simulink model "pendulum_2"  (R2013b)
settings: Solver=ode45  StartTime=0.0  StopTime=10.0  RelTol=1e-3
undefined symbols (not defined in the file or in its folder): g, l_p, l_w, m_car, v_R
settings Model: Creator=daniel  LastModifiedBy=daniel

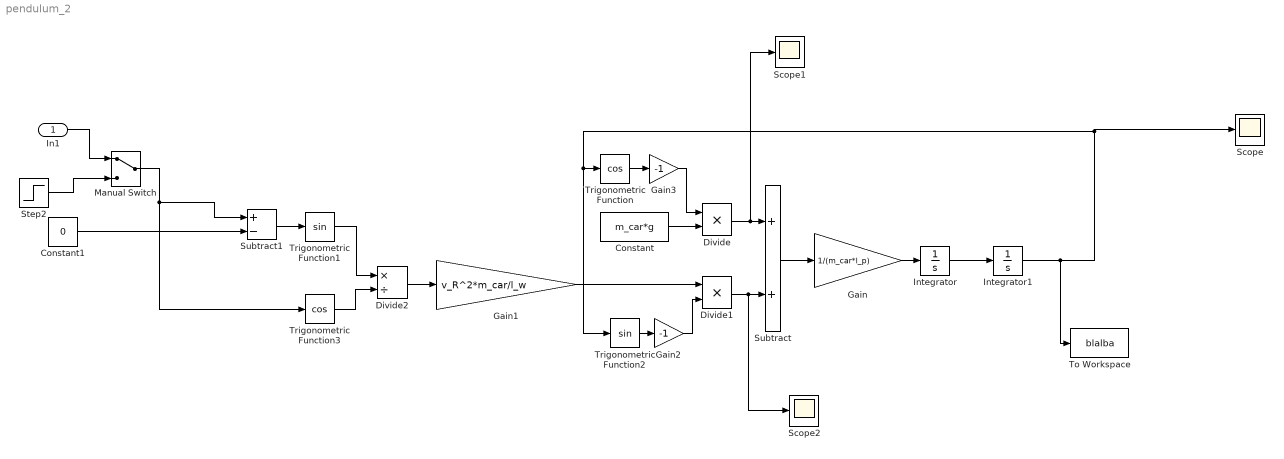
== system pendulum_2 ==
  In1 : Inport
  Constant : Constant  Value=m_car*g
  Constant1 : Constant  Value=0
  Divide : Product  Inputs=**
  Divide1 : Product  Inputs=**
  Divide2 : Product  Inputs=*/
  Gain : Gain  Gain=1/(m_car*l_p)
  Gain1 : Gain  Gain=v_R^2*m_car/l_w
  Gain2 : Gain  Gain=-1
  Gain3 : Gain  Gain=-1
  Integrator : Integrator  ContinuousStateAttributes='rho_dot'
  Integrator1 : Integrator  InitialCondition=pi/2+0.01  ContinuousStateAttributes='rho'
  Manual Switch : ManualSwitch
  Scope : Scope
  Scope1 : Scope
  Scope2 : Scope
      settings: SaveName=ScopeData2
  Step2 : Step  Time=7  After=0.8  SampleTime=0.01
  Subtract : Sum
  Subtract1 : Sum  Inputs=+-
  To Workspace : ToWorkspace  VariableName=blalba  SampleTime=-1  SaveFormat=Timeseries
  Trigonometric Function : Trigonometry  Operator=cos
  Trigonometric Function1 : Trigonometry
  Trigonometric Function2 : Trigonometry
  Trigonometric Function3 : Trigonometry  Operator=cos
  wires:
  Integrator/1 -> Integrator1/1
  Divide1/1 -> Scope2/1, Subtract/2
  Divide/1 -> Scope1/1, Subtract/1
  Manual Switch/1 -> Trigonometric Function3/1, Subtract1/1
  Constant1/1 -> Subtract1/2
  Trigonometric Function1/1 -> Divide2/1
  Trigonometric Function/1 -> Gain3/1
  Divide2/1 -> Gain1/1
  Gain/1 -> Integrator/1
  Subtract/1 -> Gain/1
  Subtract1/1 -> Trigonometric Function1/1
  Gain1/1 -> Divide1/1
  Constant/1 -> Divide/2
  Trigonometric Function3/1 -> Divide2/2
  Integrator1/1 -> To Workspace/1, Scope/1, Trigonometric Function/1, Trigonometric Function2/1
  Gain3/1 -> Divide/1
  Trigonometric Function2/1 -> Gain2/1
  Gain2/1 -> Divide1/2
  Step2/1 -> Manual Switch/2
  In1/1 -> Manual Switch/1
